simulink model "model"  (R2023a)
settings: Solver=VariableStepAuto  StartTime=0.0  StopTime=25  FixedStep=0.001  RelTol=1e-5  AbsTol=1e-5  EnableMultiTasking=on
undefined symbols (not defined in the file or in its folder): control_Q5
settings Model: Creator=pmorin  LastModifiedBy=haoyuan
settings SolverCC: AutoScaleAbsTol=off  AlgebraicLoopSolver=TrustRegion
settings DataIOCC: LimitDataPoints=on  SaveFormat=Array  SignalLoggingSaveFormat=ModelDataLogs  ReturnWorkspaceOutputs=off
settings OptimizationCC: BooleanDataType=off  ExpressionDepthLimit=2147483647  LifeSpan=inf
settings DebuggingCC: SaveWithParameterizedLinksMsg=none  UnderspecifiedInitializationDetection=Classic  MergeDetectMultiDrivingBlocksExec=none  SignalResolutionControl=TryResolveAllWithWarning  MultiTaskDSMMsg=warning  MultiTaskCondExecSysMsg=none  FcnCallInpInsideContextMsg=warning  UnconnectedInputMsg=warning  UnconnectedOutputMsg=warning  UnconnectedLineMsg=warning  StateNameClashWarn=warning  SFUnexpectedBacktrackingDiag=warning  SFNoUnconditionalDefaultTransitionDiag=warning  SFExecutionAtInitializationDiag=none  ArithmeticOperatorsInVariantConditions=warning
settings HardwareCC: ProdBitPerPointer=32  ProdBitPerSizeT=32  ProdBitPerPtrDiffT=32  ProdLargestAtomicFloat=None  ProdIntDivRoundTo=Undefined  ProdEndianess=Unspecified  ProdWordSize=32  ProdHWDeviceType=32-bit Generic  TargetUnknown=on
settings ModelReferenceCC: EnableRefExpFcnMdlSchedulingChecks=on  PropagateSignalLabelsOutOfModel=off
settings SFSimCC: SimUseLocalCustomCode=off  CustomCodeUndefinedFunction=UseInterfaceOnly
settings RTWCC: RTWUseLocalCustomCode=off
settings CodeAppCC: StateflowObjectComments=on
settings GRTTargetCC: TargetLangStandard=C89/C90 (ANSI)  CombineOutputUpdateFcns=off  GRTInterface=on
settings ConfigComp: CovMetricSettings=dw  CovSaveCumulativeToWorkspaceVar=on  CovSaveSingleToWorkspaceVar=on  CovExternalEMLEnable=off

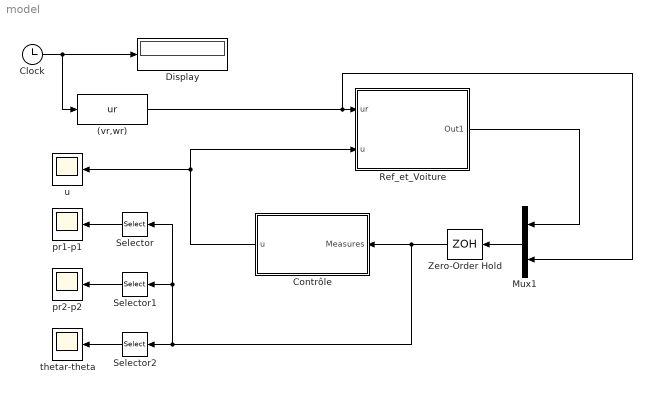
== system model ==
  (vr,wr) : MATLABFcn  MATLABFcn=ur  OutputDimensions=2
  Clock : Clock
  Contrôle : Subsystem  TreatAsAtomicUnit=on
  Display : Display
  Mux1 : Mux  Inputs=2
  Ref_et_Voiture : Subsystem  mask{init=[0;0;0;2;5;0.1/4*pi;0]}
      mask prompts: init "Initial values"
  Selector : Selector  InputPortWidth=9  IndexOptions=Index vector (dialog)  Indices=[1 4]  OutputSizes=1
  Selector1 : Selector  InputPortWidth=9  IndexOptions=Index vector (dialog)  Indices=[2 5]  OutputSizes=1
  Selector2 : Selector  InputPortWidth=9  IndexOptions=Index vector (dialog)  Indices=[3 6]  OutputSizes=1
  Zero-Order Hold : ZeroOrderHold  SampleTime=0.0001
  pr1-p1 : Scope
  pr2-p2 : Scope
  thetar-theta : Scope
  u : Scope
  wires:
  Clock/1 -> (vr,wr)/1, Display/1
  Ref_et_Voiture/1(Out1) -> Mux1/1
  Contrôle/1(u) -> Ref_et_Voiture/2(u), u/1
  Mux1/1 -> Zero-Order Hold/1
  Zero-Order Hold/1 -> Selector1/1, Selector/1, Selector2/1, Contrôle/1(Measures)
  Selector/1 -> pr1-p1/1
  Selector1/1 -> pr2-p2/1
  Selector2/1 -> thetar-theta/1
  (vr,wr)/1 -> Mux1/2, Ref_et_Voiture/1(ur)

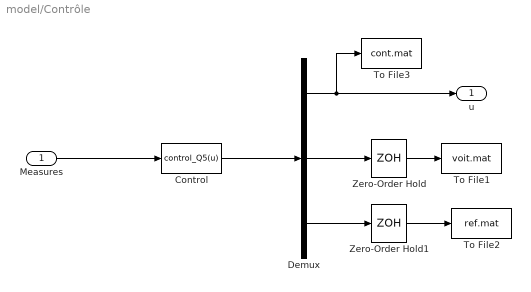
== system model/Contrôle ==
  Measures : Inport
  Control : MATLABFcn  MATLABFcn=control_Q5(u)  OutputDimensions=9
  Demux : Demux  Outputs=[2 4 3]
      settings: DisplayOption=none
  To File1 : ToFile  Filename=voit.mat
  To File2 : ToFile  Filename=ref.mat
  To File3 : ToFile  Filename=cont.mat
  Zero-Order Hold : ZeroOrderHold  SampleTime=-1
  Zero-Order Hold1 : ZeroOrderHold  SampleTime=-1
  u : Outport  VectorParamsAs1DForOutWhenUnconnected=off
  wires:
  Zero-Order Hold/1 -> To File1/1
  Demux/3 -> Zero-Order Hold1/1
  Demux/2 -> Zero-Order Hold/1
  Demux/1 -> u/1, To File3/1
  Measures/1 -> Control/1
  Control/1 -> Demux/1
  Zero-Order Hold1/1 -> To File2/1

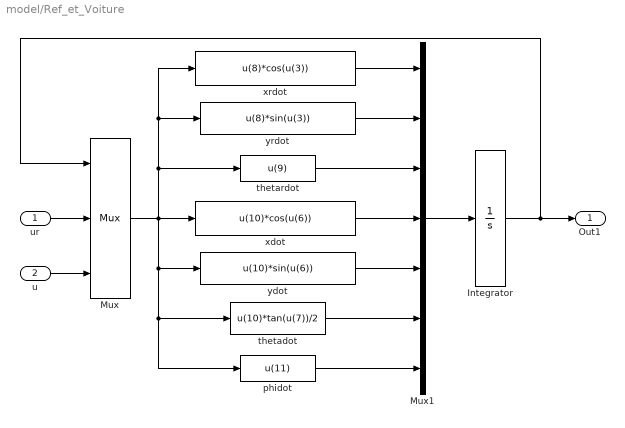
== system model/Ref_et_Voiture ==
  ur : Inport
  u : Inport  Port=2
  Integrator : Integrator  InitialCondition=init
  Mux : Mux  Inputs=[7 2 2]
  Mux1 : Mux  Inputs=7
  phidot : Fcn  Expr=u(11)
  thetadot : Fcn  Expr=u(10)*tan(u(7))/2
  thetardot : Fcn  Expr=u(9)
  xdot : Fcn  Expr=u(10)*cos(u(6))
  xrdot : Fcn  Expr=u(8)*cos(u(3))
  ydot : Fcn  Expr=u(10)*sin(u(6))
  yrdot : Fcn  Expr=u(8)*sin(u(3))
  Out1 : Outport  VectorParamsAs1DForOutWhenUnconnected=off
  wires:
  ur/1 -> Mux/2
  Integrator/1 -> Out1/1, Mux/1
  Mux1/1 -> Integrator/1
  Mux/1 -> thetardot/1, yrdot/1, xrdot/1, ydot/1, thetadot/1, phidot/1, xdot/1
  u/1 -> Mux/3
  phidot/1 -> Mux1/7
  thetadot/1 -> Mux1/6
  ydot/1 -> Mux1/5
  xdot/1 -> Mux1/4
  thetardot/1 -> Mux1/3
  xrdot/1 -> Mux1/1
  yrdot/1 -> Mux1/2
